simulink model "MostionDetection1_Edge"  (R2016a)
settings: Solver=VariableStepAuto  StartTime=0.0  StopTime=inf  RelTol=1e-3
undefined symbols (not defined in the file): none, videoinput
libraries: visionstatistics x1, simulink x1, visiontextngfix x1, visionanalysis x1, imaqlib x1
settings Model: Creator=YASARA  LastModifiedBy=YASARA

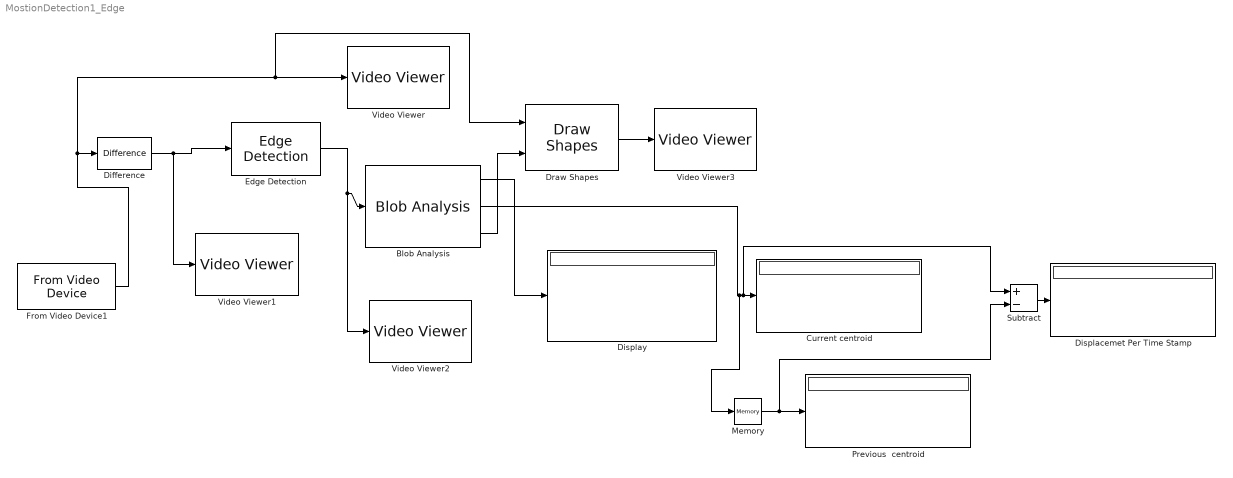
== system MostionDetection1_Edge ==
  Blob Analysis : visionstatistics/Blob Analysis  Tag=vipblks_row_conv  area=on  centroid=on  bBox=on  majorAxis=off  minorAxis=off  angle=off  eccentricity=off  equivDiameterSq=off  extent=off  perimeter=off  maxBlobs=1  warnIfNumBlobsExceeded=on  isCount=off  useMinArea=off  minArea=0  useMaxArea=off  maxArea=intmax('uint32')  excludeBorderBlob=off  outDT=double  isOutVarDim=off  isFill=on  fillValues=-1  conn=4  isLabel=off  outputMode=Binary point scaling  outputWordLength=32  outputFracLength=16  firstCoeffMode=Binary point scaling  firstCoeffWordLength=16  firstCoeffFracLength=14  secondCoeffMode=Binary point scaling  secondCoeffWordLength=32  secondCoeffFracLength=16  accumMode=Binary point scaling  accumWordLength=32  accumFracLength=0  prodOutputMode=Binary point scaling  prodOutputWordLength=32  prodOutputFracLength=16  roundingMode=Floor  overflowMode=off
  Current centroid : Display
  Difference : simulink/Discrete/Difference  ICPrevInput=0.0  OutMin=[]  OutMax=[]  OutDataType=fixdt(1, 16)  OutScaling=2^-10  DoSatur=off
  Displacemet Per Time Stamp : Display
  Display : Display
  Draw Shapes : visiontextngfix/Draw Shapes  shape=Rectangles  fill=off  lineWidth=1  fillClrSource=Specify via dialog  display=Black  intensity=200  color=[200 255 100]  opacity=0.6  viewport=Entire image  antialiasing=off  inType=Obsolete  imagePorts=One multidimensional signal  prodOutputMode=Binary point scaling  prodOutputWordLength=32  prodOutputFracLength=14  memoryMode=Specify word length  memoryWordLength=16  memoryFracLength=15  roundingMode=Floor  overflowMode=off
  Edge Detection : visionanalysis/Edge Detection  method=Prewitt  outputType=Binary image  userDefinedThreshold=off  thresholdSource=Input port  threshold=20  thresholdTuning=4  edgeThinning=off  threshold_canny=[0.25 0.60]  autoPercent=70  sigma=1  prodOutputMode=Binary point scaling  prodOutputWordLength=32  prodOutputFracLength=8  roundingMode=Floor  overflowMode=off
  From Video Device1 : imaqlib/From Video Device  DeviceMenu=winvideo 2 (USB Video Device)  Device=winvideo 2 (USB Video Device)  ObjConstructor=videoinput('winvideo', 2)  VideoFormatMenu=YUY2_160x120  VideoFormat=YUY2_160x120  VideoSource=input1  ROIPosition=[0 0 120 160]  EnableHWTrigger=off  TriggerConfiguration=none/none  SampleTime=1/30  OutputPortsMode=One multidimensional signal  DataType=single  CanDoHWTrigger=no  ReturnedColorSpace=grayscale  BlockHandle=154.0001  ROIWidth=160  ROIHeight=120  ROIColumn=0  ROIRow=0  EngXMLPath=C:\Program Files\MATLAB\R2016a\toolbox\imaq\imaq\private  DevXMLPath=C:\MATLAB\SupportPackages\R2016a\toolbox\imaq\supportpackages\genericvideo\adaptor\win64  EngLibPath=C:\Program Files\MATLAB\R2016a\toolbox\imaq\imaqblks\imaqmex\win64  ColorSpace=grayscale  BayerSensorAlignment=grbg
  Memory : Memory  InheritSampleTime=on
  Previous  centroid : Display
  Subtract : Sum  Inputs=+-
  Video Viewer : VideoViewer  FigPos=[2 408 410 300]
  Video Viewer1 : VideoViewer  FigPos=[-77 1306 1362 626]
  Video Viewer2 : VideoViewer  FigPos=[853 419 410 300]
  Video Viewer3 : VideoViewer  FigPos=[54 586 412 300]
  wires:
  From Video Device1/1 -> Draw Shapes/1, Video Viewer/1, Difference/1
  Difference/1 -> Video Viewer1/1, Edge Detection/1
  Edge Detection/1 -> Video Viewer2/1, Blob Analysis/1
  Draw Shapes/1 -> Video Viewer3/1
  Blob Analysis/1 -> Display/1
  Blob Analysis/3 -> Draw Shapes/2
  Memory/1 -> Subtract/2, Previous  centroid/1
  Blob Analysis/2 -> Memory/1, Subtract/1, Current centroid/1
  Subtract/1 -> Displacemet Per Time Stamp/1
